simulink model "simulation_prev"  (R2021b)
settings: Solver=ode45  StartTime=0.0  StopTime=20.0  RelTol=1e-3
model workspace (MAT data in the model file):
  instants = 1
values from neighbouring files (symbols this model uses):
  c = modNE(x2,x2,e0,m,I,A,pc)    [ct_dynamics.m]    (also in dynamic_model_3R_spatial.m = [c1;c2;c3]; dynamic_model_simulation.m = [0.4; 0.2; 0.7]; run_experiment.m = [0.4; 0.2; 0.7])
  c0bar = norm(get_c_factorization_matrix(sol(1),sol(2),sol(3),sol(4),sol(5)))/norm(sol(3:5))    [compute_vel_obs_gain.m]    (also in dynamic_model_simulation.m = 1.96239028072; red_obs_gain_computation.m = c0; run_experiment.m = 1.96239028072)
  DHTABLE = [ pi/2      0         l(1)     q1 ... (first row only)    [compute_vel_obs_gain.m]    (also in dynamic_model_3R_spatial.m = [ pi/2      0      sym('L1') sym('q1'); dynamic_model_simulation.m = [ pi/2      0         l(1)     0; red_obs_gain_computation.m = [ pi/2      0         l(1)     0; run_experiment.m = [ pi/2      0         l(1)     0)
  eta = 1    [compute_vel_obs_gain.m]    (also in dynamic_model_simulation.m; red_obs_gain_computation.m; run_experiment.m)
  g0 = 9.81    [compute_vel_obs_gain.m]    (also in dynamic_model_3R_spatial.m; dynamic_model_simulation.m; modNE.m = 0; red_obs_gain_computation.m)
  I = zeros(3,3,N)    [compute_vel_obs_gain.m]    (also in dynamic_model_simulation.m; red_obs_gain_computation.m; run_experiment.m; run_simulation.m = zeros(3,3,3))
  K0 = c0bar*(v_max+eta)/(2*lambda_1)    [compute_vel_obs_gain.m]    (also in dynamic_model_simulation.m = 31.0539244645; red_obs_gain_computation.m = 0; run_experiment.m = 103.513081548)
  Kd = 3e1    (= 30)    [dynamic_model_simulation.m]    (also in run_experiment.m = 70; run_simulation.m = 10)
  Ko = 5e1    (= 50)    [dynamic_model_simulation.m]    (also in run_experiment.m; run_simulation.m = 0.1)
  Kp = 3e2    (= 300)    [dynamic_model_simulation.m]    (also in run_experiment.m = 70; run_simulation.m = 50)
  l = [0.5 0.5 0.4]'    [compute_eeJacobian.m]    (also in compute_vel_obs_gain.m; dynamic_model_simulation.m; eeJacobian_3R_spatial.m; red_obs_gain_computation.m)
  lambda_1 = min(min_first,min_third)/2    [compute_vel_obs_gain.m]    (also in dynamic_model_simulation.m = 0.0947894822263; red_obs_gain_computation.m = min_eig/2; run_experiment.m = 0.0473947411131)
  m = [15 10 5]'    [compute_vel_obs_gain.m]    (also in dynamic_model_simulation.m; red_obs_gain_computation.m; run_experiment.m; run_simulation.m = [m1 m2 m3]')
  pc = [0             -l(2)+dc(2) -l(3)+dc(3) ... (first row only)    [compute_vel_obs_gain.m]    (also in dynamic_model_simulation.m; red_obs_gain_computation.m; run_experiment.m)
  q0 = inverse_kinematics(p_init,l,soln_type)    [dynamic_model_simulation.m]    (also in run_experiment.m; run_simulation.m = [0,0,0]')
  r_c = 0.3    [dynamic_model_simulation.m]    (also in run_experiment.m)
  s0 = ceil(norm(dq0)/vbar)    [dynamic_model_simulation.m]
  T = simplify(T)    [DHMatrix.m]    (also in DHMatrix_sym.m; dynamic_model_3R_spatial.m = simplify(T1+T2+T3); dynamic_model_simulation.m = 2; run_experiment.m = 2)
  t0 = 2    [dynamic_model_simulation.m]    (also in run_experiment.m)
  T0 = 0.5*x2hat0'*M0*x2hat0    [dynamic_model_simulation.m]    (also in run_experiment.m)
  vbar = 2*eta+1    (= 3)    [dynamic_model_simulation.m]
  x0 = [pi/4,pi/4,1,1,1]'    [compute_vel_obs_gain.m]    (also in dynamic_model_simulation.m = [q0; dq0]; find_c0.m; run_experiment.m = [q0; dq0])
  z0 = [0 0 1]'    [dynamic_model_3R_spatial.m]    (also in dynamic_model_simulation.m = x2hat0 - K0*q0; run_experiment.m = x2hat0 - K0*q0)
undefined symbols (not defined in the file or in its folder): Levenberg, Marquardt, p_f, p_i, t_fin, t_init, time_int, trvec2tform
libraries: robotcorelib x3, SignalEditorBlockLib x1, robotmaniplib x1, matrix_library x1
(part 2 of 2)

== matlab function simulation_prev/reduced observer implementation/energy residual/MATLAB Function5 ==
  data: arrays input; T output; A output
function [T, A] = DHMatrix(arrays)
% T = DHMatrix(arrays) takes as inputs:
%   -arrays: a n-vector of vectors composed like this: [alpha a d theta]
% and outputs:
%   -T: the product of all the matrices corresponding to each vector of arrays
% Remember that:
% cos(q1 + q2) = cos(q1)*cos(q2) - sin(q1)*sin(q2)
% sin(q1 + q2) = cos(q1)*sin(q2) + cos(q2)*sin(q1)
% making use of the simplify function these are converted automatically

    T = eye(4);
    nums = size(arrays);
    
    A = zeros(4,4,nums(1));
    
    for i = 1:nums(1)
        line = arrays(i, :);
        R = [cos(line(4)) -cos(line(1))*sin(line(4)) sin(line(1))*sin(line(4)) line(2)*cos(line(4));
             sin(line(4)) cos(line(1))*cos(line(4)) -sin(line(1))*cos(line(4)) line(2)*sin(line(4));
             0 sin(line(1)) cos(line(1)) line(3);
             0 0 0 1];
        A(:,:,i) = R;
        T = T * R;   
    end
end

== matlab function simulation_prev/reduced observer implementation/energy residual/MATLAB Function6 ==
  data: dq input; u output; v input; ddq input; m input; I input; A input; pc input; g0 input
function u = modNE(dq,v,ddq,m,I,A,pc,g0)
% Implementation of Modified Newton-Euler algorithm

n = size(dq,1);
% check dimension consistency
if ~(size(v,1)==n && size(ddq,1)==n && size(dq,2)==1 && ...
     size(v,2)==1 && size(ddq,2)==1 && size(m,1)==n && ...
     size(I,3)==n && size(A,3)==n && size(pc,2)==n) 
    disp("Inconsistent input arguments dimension")
    u = zeros(n,1);
    return
end

% initialization
R = A(1:3,1:3,:);
p = [R(:,:,1)'*A(1:3,4,1) R(:,:,2)'*A(1:3,4,2) R(:,:,3)'*A(1:3,4,3)];
w = zeros(3,n+1);
wa = zeros(3,n+1);
dw = zeros(3,n+1);
a = zeros(3,n+1)-[[0 0 -g0]' zeros(3,n)];
ac = zeros(3,n+1);
f = zeros(3,n+1);
t = zeros(3,n+1);
u = zeros(n,1);

% forward recursion
for i = 2:n+1
   w(:,i) = R(:,:,i-1)'*(w(:,i-1)+dq(i-1)*[0 0 1]');
   wa(:,i) = R(:,:,i-1)'*(wa(:,i-1)+v(i-1)*[0 0 1]');
   dw(:,i) = R(:,:,i-1)'*(dw(:,i-1)+ddq(i-1)*[0 0 1]'+cross(dq(i-1)*wa(:,i-1),[0 0 1]'));
   a(:,i) = R(:,:,i-1)'*a(:,i-1)+cross(dw(:,i),p(:,i-1))+cross(w(:,i),cross(wa(:,i),p(:,i-1)));
   ac(:,i) = a(:,i)+cross(dw(:,i),pc(:,i-1))+cross(w(:,i),cross(wa(:,i),pc(:,i-1)));
end

w = w(:,2:n+1);
wa = wa(:,2:n+1);
dw = dw(:,2:n+1);
ac = ac(:,2:n+1);
R = cat(3,R,eye(3));

% backward recursion
for i = n:-1:1
    f(:,i) = R(:,:,i+1)*f(:,i+1)+m(i)*ac(:,i);
    t(:,i) = R(:,:,i+1)*t(:,i+1)+cross(R(:,:,i+1)*f(:,i+1),pc(:,i))-cross(f(:,i),p(:,i)+pc(:,i))+I(:,:,i)*dw(:,i)+cross(w(:,i),I(:,:,i)*wa(:,i));
    % assuming all revolute joints
    u(i) = t(:,i)'*(R(:,:,i)'*[0 0 1]');
end
end

== matlab function simulation_prev/reduced observer implementation/observer dynamics/MATLAB Function1 ==
  data: x2hat input; s input; vbar input; eta input; next_s output
function next_s = s_dynamics(x2hat,s,vbar,eta)
norm_x2hat = norm(x2hat);
if ((norm_x2hat >= s*vbar-eta) && ~(norm_x2hat <= s*vbar+eta))
    next_s = s+1;
elseif ((norm_x2hat <= (s-1)*vbar+eta) && ~(norm_x2hat >= (s-1)*vbar-eta) && s~=1)
    next_s = s-1;
else
    next_s = s;
end
end

== matlab function simulation_prev/finite differentiation/Controller/MATLAB Function1 ==
  data: dq input; u output; v input; ddq input; m input; I input; A input; pc input; g0 input
function u = modNE(dq,v,ddq,m,I,A,pc,g0)
% Implementation of Modified Newton-Euler algorithm

n = size(dq,1);
% check dimension consistency
if ~(size(v,1)==n && size(ddq,1)==n && size(dq,2)==1 && ...
     size(v,2)==1 && size(ddq,2)==1 && size(m,1)==n && ...
     size(I,3)==n && size(A,3)==n && size(pc,2)==n) 
    disp("Inconsistent input arguments dimension")
    u = zeros(n,1);
    return
end

% initialization
R = A(1:3,1:3,:);
p = [R(:,:,1)'*A(1:3,4,1) R(:,:,2)'*A(1:3,4,2) R(:,:,3)'*A(1:3,4,3)];
w = zeros(3,n+1);
wa = zeros(3,n+1);
dw = zeros(3,n+1);
a = zeros(3,n+1)-[[0 0 -g0]' zeros(3,n)];
ac = zeros(3,n+1);
f = zeros(3,n+1);
t = zeros(3,n+1);
u = zeros(n,1);

% forward recursion
for i = 2:n+1
   w(:,i) = R(:,:,i-1)'*(w(:,i-1)+dq(i-1)*[0 0 1]');
   wa(:,i) = R(:,:,i-1)'*(wa(:,i-1)+v(i-1)*[0 0 1]');
   dw(:,i) = R(:,:,i-1)'*(dw(:,i-1)+ddq(i-1)*[0 0 1]'+cross(dq(i-1)*wa(:,i-1),[0 0 1]'));
   a(:,i) = R(:,:,i-1)'*a(:,i-1)+cross(dw(:,i),p(:,i-1))+cross(w(:,i),cross(wa(:,i),p(:,i-1)));
   ac(:,i) = a(:,i)+cross(dw(:,i),pc(:,i-1))+cross(w(:,i),cross(wa(:,i),pc(:,i-1)));
end

w = w(:,2:n+1);
wa = wa(:,2:n+1);
dw = dw(:,2:n+1);
ac = ac(:,2:n+1);
R = cat(3,R,eye(3));

% backward recursion
for i = n:-1:1
    f(:,i) = R(:,:,i+1)*f(:,i+1)+m(i)*ac(:,i);
    t(:,i) = R(:,:,i+1)*t(:,i+1)+cross(R(:,:,i+1)*f(:,i+1),pc(:,i))-cross(f(:,i),p(:,i)+pc(:,i))+I(:,:,i)*dw(:,i)+cross(w(:,i),I(:,:,i)*wa(:,i));
    % assuming all revolute joints
    u(i) = t(:,i)'*(R(:,:,i)'*[0 0 1]');
end
end

== matlab function simulation_prev/finite differentiation/Controller/MATLAB Function3 ==
  data: arrays input; T output; A output
function [T, A] = DHMatrix(arrays)
% T = DHMatrix(arrays) takes as inputs:
%   -arrays: a n-vector of vectors composed like this: [alpha a d theta]
% and outputs:
%   -T: the product of all the matrices corresponding to each vector of arrays
% Remember that:
% cos(q1 + q2) = cos(q1)*cos(q2) - sin(q1)*sin(q2)
% sin(q1 + q2) = cos(q1)*sin(q2) + cos(q2)*sin(q1)
% making use of the simplify function these are converted automatically

    T = eye(4);
    nums = size(arrays);
    
    A = zeros(4,4,nums(1));
    
    for i = 1:nums(1)
        line = arrays(i, :);
        R = [cos(line(4)) -cos(line(1))*sin(line(4)) sin(line(1))*sin(line(4)) line(2)*cos(line(4));
             sin(line(4)) cos(line(1))*cos(line(4)) -sin(line(1))*cos(line(4)) line(2)*sin(line(4));
             0 sin(line(1)) cos(line(1)) line(3);
             0 0 0 1];
        A(:,:,i) = R;
        T = T * R;   
    end
end

== matlab function simulation_prev/finite differentiation/Robot dynamics/MATLAB Function ==
  data: x input; u input; dx output; m input; I input; A input; pc input; g0 input
function dx = ct_dynamics(x,u,m,I,A,pc,g0)
% return the continuous time dynamics given state and input
e0 = zeros(3,1);
e1 = [1 0 0]';
e2 = [0 1 0]';
e3 = [0 0 1]';
x2 = x(4:6);
%get inertia matrix M from modNE algorithm
M = [modNE(e0,e0,e1,m,I,A,pc,0) modNE(e0,e0,e2,m,I,A,pc,0) modNE(e0,e0,e3,m,I,A,pc,0)];
iM = inv(M);
cg =  modNE(x2,x2,e0,m,I,A,pc,g0);
dx=[x2;
    iM*(-cg+u)];
end

== matlab function simulation_prev/finite differentiation/Robot dynamics/MATLAB Function2 ==
  data: arrays input; T output; A output
function [T, A] = DHMatrix(arrays)
% T = DHMatrix(arrays) takes as inputs:
%   -arrays: a n-vector of vectors composed like this: [alpha a d theta]
% and outputs:
%   -T: the product of all the matrices corresponding to each vector of arrays
% Remember that:
% cos(q1 + q2) = cos(q1)*cos(q2) - sin(q1)*sin(q2)
% sin(q1 + q2) = cos(q1)*sin(q2) + cos(q2)*sin(q1)
% making use of the simplify function these are converted automatically

    T = eye(4);
    nums = size(arrays);
    
    A = zeros(4,4,nums(1));
    
    for i = 1:nums(1)
        line = arrays(i, :);
        R = [cos(line(4)) -cos(line(1))*sin(line(4)) sin(line(1))*sin(line(4)) line(2)*cos(line(4));
             sin(line(4)) cos(line(1))*cos(line(4)) -sin(line(1))*cos(line(4)) line(2)*sin(line(4));
             0 sin(line(1)) cos(line(1)) line(3);
             0 0 0 1];
        A(:,:,i) = R;
        T = T * R;   
    end
end

== matlab function simulation_prev/full state implementation/Robot dynamics/MATLAB Function ==
  data: x input; u input; dx output; m input; I input; A input; pc input; g0 input
function dx = ct_dynamics(x,u,m,I,A,pc,g0)
% return the continuous time dynamics given state and input
e0 = zeros(3,1);
e1 = [1 0 0]';
e2 = [0 1 0]';
e3 = [0 0 1]';
x2 = x(4:6);
%get inertia matrix M from modNE algorithm
M = [modNE(e0,e0,e1,m,I,A,pc,0) modNE(e0,e0,e2,m,I,A,pc,0) modNE(e0,e0,e3,m,I,A,pc,0)];
cg =  modNE(x2,x2,e0,m,I,A,pc,g0);
dx=[x2;
    inv(M)*(-cg+u)];
end

== matlab function simulation_prev/finite differentiation/energy residual/MATLAB Function2 ==
  data: dq input; u output; v input; ddq input; m input; I input; A input; pc input; g0 input
function u = modNE(dq,v,ddq,m,I,A,pc,g0)
% Implementation of Modified Newton-Euler algorithm

n = size(dq,1);
% check dimension consistency
if ~(size(v,1)==n && size(ddq,1)==n && size(dq,2)==1 && ...
     size(v,2)==1 && size(ddq,2)==1 && size(m,1)==n && ...
     size(I,3)==n && size(A,3)==n && size(pc,2)==n) 
    disp("Inconsistent input arguments dimension")
    u = zeros(n,1);
    return
end

% initialization
R = A(1:3,1:3,:);
p = [R(:,:,1)'*A(1:3,4,1) R(:,:,2)'*A(1:3,4,2) R(:,:,3)'*A(1:3,4,3)];
w = zeros(3,n+1);
wa = zeros(3,n+1);
dw = zeros(3,n+1);
a = zeros(3,n+1)-[[0 0 -g0]' zeros(3,n)];
ac = zeros(3,n+1);
f = zeros(3,n+1);
t = zeros(3,n+1);
u = zeros(n,1);

% forward recursion
for i = 2:n+1
   w(:,i) = R(:,:,i-1)'*(w(:,i-1)+dq(i-1)*[0 0 1]');
   wa(:,i) = R(:,:,i-1)'*(wa(:,i-1)+v(i-1)*[0 0 1]');
   dw(:,i) = R(:,:,i-1)'*(dw(:,i-1)+ddq(i-1)*[0 0 1]'+cross(dq(i-1)*wa(:,i-1),[0 0 1]'));
   a(:,i) = R(:,:,i-1)'*a(:,i-1)+cross(dw(:,i),p(:,i-1))+cross(w(:,i),cross(wa(:,i),p(:,i-1)));
   ac(:,i) = a(:,i)+cross(dw(:,i),pc(:,i-1))+cross(w(:,i),cross(wa(:,i),pc(:,i-1)));
end

w = w(:,2:n+1);
wa = wa(:,2:n+1);
dw = dw(:,2:n+1);
ac = ac(:,2:n+1);
R = cat(3,R,eye(3));

% backward recursion
for i = n:-1:1
    f(:,i) = R(:,:,i+1)*f(:,i+1)+m(i)*ac(:,i);
    t(:,i) = R(:,:,i+1)*t(:,i+1)+cross(R(:,:,i+1)*f(:,i+1),pc(:,i))-cross(f(:,i),p(:,i)+pc(:,i))+I(:,:,i)*dw(:,i)+cross(w(:,i),I(:,:,i)*wa(:,i));
    % assuming all revolute joints
    u(i) = t(:,i)'*(R(:,:,i)'*[0 0 1]');
end
end

== matlab function simulation_prev/finite differentiation/energy residual/MATLAB Function3 ==
  data: dq input; u output; v input; ddq input; m input; I input; A input; pc input; g0 input
function u = modNE(dq,v,ddq,m,I,A,pc,g0)
% Implementation of Modified Newton-Euler algorithm

n = size(dq,1);
% check dimension consistency
if ~(size(v,1)==n && size(ddq,1)==n && size(dq,2)==1 && ...
     size(v,2)==1 && size(ddq,2)==1 && size(m,1)==n && ...
     size(I,3)==n && size(A,3)==n && size(pc,2)==n) 
    disp("Inconsistent input arguments dimension")
    u = zeros(n,1);
    return
end

% initialization
R = A(1:3,1:3,:);
p = [R(:,:,1)'*A(1:3,4,1) R(:,:,2)'*A(1:3,4,2) R(:,:,3)'*A(1:3,4,3)];
w = zeros(3,n+1);
wa = zeros(3,n+1);
dw = zeros(3,n+1);
a = zeros(3,n+1)-[[0 0 -g0]' zeros(3,n)];
ac = zeros(3,n+1);
f = zeros(3,n+1);
t = zeros(3,n+1);
u = zeros(n,1);

% forward recursion
for i = 2:n+1
   w(:,i) = R(:,:,i-1)'*(w(:,i-1)+dq(i-1)*[0 0 1]');
   wa(:,i) = R(:,:,i-1)'*(wa(:,i-1)+v(i-1)*[0 0 1]');
   dw(:,i) = R(:,:,i-1)'*(dw(:,i-1)+ddq(i-1)*[0 0 1]'+cross(dq(i-1)*wa(:,i-1),[0 0 1]'));
   a(:,i) = R(:,:,i-1)'*a(:,i-1)+cross(dw(:,i),p(:,i-1))+cross(w(:,i),cross(wa(:,i),p(:,i-1)));
   ac(:,i) = a(:,i)+cross(dw(:,i),pc(:,i-1))+cross(w(:,i),cross(wa(:,i),pc(:,i-1)));
end

w = w(:,2:n+1);
wa = wa(:,2:n+1);
dw = dw(:,2:n+1);
ac = ac(:,2:n+1);
R = cat(3,R,eye(3));

% backward recursion
for i = n:-1:1
    f(:,i) = R(:,:,i+1)*f(:,i+1)+m(i)*ac(:,i);
    t(:,i) = R(:,:,i+1)*t(:,i+1)+cross(R(:,:,i+1)*f(:,i+1),pc(:,i))-cross(f(:,i),p(:,i)+pc(:,i))+I(:,:,i)*dw(:,i)+cross(w(:,i),I(:,:,i)*wa(:,i));
    % assuming all revolute joints
    u(i) = t(:,i)'*(R(:,:,i)'*[0 0 1]');
end
end

== matlab function simulation_prev/finite differentiation/energy residual/MATLAB Function4 ==
  data: dq input; u output; v input; ddq input; m input; I input; A input; pc input; g0 input
function u = modNE(dq,v,ddq,m,I,A,pc,g0)
% Implementation of Modified Newton-Euler algorithm

n = size(dq,1);
% check dimension consistency
if ~(size(v,1)==n && size(ddq,1)==n && size(dq,2)==1 && ...
     size(v,2)==1 && size(ddq,2)==1 && size(m,1)==n && ...
     size(I,3)==n && size(A,3)==n && size(pc,2)==n) 
    disp("Inconsistent input arguments dimension")
    u = zeros(n,1);
    return
end

% initialization
R = A(1:3,1:3,:);
p = [R(:,:,1)'*A(1:3,4,1) R(:,:,2)'*A(1:3,4,2) R(:,:,3)'*A(1:3,4,3)];
w = zeros(3,n+1);
wa = zeros(3,n+1);
dw = zeros(3,n+1);
a = zeros(3,n+1)-[[0 0 -g0]' zeros(3,n)];
ac = zeros(3,n+1);
f = zeros(3,n+1);
t = zeros(3,n+1);
u = zeros(n,1);

% forward recursion
for i = 2:n+1
   w(:,i) = R(:,:,i-1)'*(w(:,i-1)+dq(i-1)*[0 0 1]');
   wa(:,i) = R(:,:,i-1)'*(wa(:,i-1)+v(i-1)*[0 0 1]');
   dw(:,i) = R(:,:,i-1)'*(dw(:,i-1)+ddq(i-1)*[0 0 1]'+cross(dq(i-1)*wa(:,i-1),[0 0 1]'));
   a(:,i) = R(:,:,i-1)'*a(:,i-1)+cross(dw(:,i),p(:,i-1))+cross(w(:,i),cross(wa(:,i),p(:,i-1)));
   ac(:,i) = a(:,i)+cross(dw(:,i),pc(:,i-1))+cross(w(:,i),cross(wa(:,i),pc(:,i-1)));
end

w = w(:,2:n+1);
wa = wa(:,2:n+1);
dw = dw(:,2:n+1);
ac = ac(:,2:n+1);
R = cat(3,R,eye(3));

% backward recursion
for i = n:-1:1
    f(:,i) = R(:,:,i+1)*f(:,i+1)+m(i)*ac(:,i);
    t(:,i) = R(:,:,i+1)*t(:,i+1)+cross(R(:,:,i+1)*f(:,i+1),pc(:,i))-cross(f(:,i),p(:,i)+pc(:,i))+I(:,:,i)*dw(:,i)+cross(w(:,i),I(:,:,i)*wa(:,i));
    % assuming all revolute joints
    u(i) = t(:,i)'*(R(:,:,i)'*[0 0 1]');
end
end

== matlab function simulation_prev/finite differentiation/energy residual/MATLAB Function5 ==
  data: arrays input; T output; A output
function [T, A] = DHMatrix(arrays)
% T = DHMatrix(arrays) takes as inputs:
%   -arrays: a n-vector of vectors composed like this: [alpha a d theta]
% and outputs:
%   -T: the product of all the matrices corresponding to each vector of arrays
% Remember that:
% cos(q1 + q2) = cos(q1)*cos(q2) - sin(q1)*sin(q2)
% sin(q1 + q2) = cos(q1)*sin(q2) + cos(q2)*sin(q1)
% making use of the simplify function these are converted automatically

    T = eye(4);
    nums = size(arrays);
    
    A = zeros(4,4,nums(1));
    
    for i = 1:nums(1)
        line = arrays(i, :);
        R = [cos(line(4)) -cos(line(1))*sin(line(4)) sin(line(1))*sin(line(4)) line(2)*cos(line(4));
             sin(line(4)) cos(line(1))*cos(line(4)) -sin(line(1))*cos(line(4)) line(2)*sin(line(4));
             0 sin(line(1)) cos(line(1)) line(3);
             0 0 0 1];
        A(:,:,i) = R;
        T = T * R;   
    end
end

== matlab function simulation_prev/finite differentiation/energy residual/MATLAB Function6 ==
  data: dq input; u output; v input; ddq input; m input; I input; A input; pc input; g0 input
function u = modNE(dq,v,ddq,m,I,A,pc,g0)
% Implementation of Modified Newton-Euler algorithm

n = size(dq,1);
% check dimension consistency
if ~(size(v,1)==n && size(ddq,1)==n && size(dq,2)==1 && ...
     size(v,2)==1 && size(ddq,2)==1 && size(m,1)==n && ...
     size(I,3)==n && size(A,3)==n && size(pc,2)==n) 
    disp("Inconsistent input arguments dimension")
    u = zeros(n,1);
    return
end

% initialization
R = A(1:3,1:3,:);
p = [R(:,:,1)'*A(1:3,4,1) R(:,:,2)'*A(1:3,4,2) R(:,:,3)'*A(1:3,4,3)];
w = zeros(3,n+1);
wa = zeros(3,n+1);
dw = zeros(3,n+1);
a = zeros(3,n+1)-[[0 0 -g0]' zeros(3,n)];
ac = zeros(3,n+1);
f = zeros(3,n+1);
t = zeros(3,n+1);
u = zeros(n,1);

% forward recursion
for i = 2:n+1
   w(:,i) = R(:,:,i-1)'*(w(:,i-1)+dq(i-1)*[0 0 1]');
   wa(:,i) = R(:,:,i-1)'*(wa(:,i-1)+v(i-1)*[0 0 1]');
   dw(:,i) = R(:,:,i-1)'*(dw(:,i-1)+ddq(i-1)*[0 0 1]'+cross(dq(i-1)*wa(:,i-1),[0 0 1]'));
   a(:,i) = R(:,:,i-1)'*a(:,i-1)+cross(dw(:,i),p(:,i-1))+cross(w(:,i),cross(wa(:,i),p(:,i-1)));
   ac(:,i) = a(:,i)+cross(dw(:,i),pc(:,i-1))+cross(w(:,i),cross(wa(:,i),pc(:,i-1)));
end

w = w(:,2:n+1);
wa = wa(:,2:n+1);
dw = dw(:,2:n+1);
ac = ac(:,2:n+1);
R = cat(3,R,eye(3));

% backward recursion
for i = n:-1:1
    f(:,i) = R(:,:,i+1)*f(:,i+1)+m(i)*ac(:,i);
    t(:,i) = R(:,:,i+1)*t(:,i+1)+cross(R(:,:,i+1)*f(:,i+1),pc(:,i))-cross(f(:,i),p(:,i)+pc(:,i))+I(:,:,i)*dw(:,i)+cross(w(:,i),I(:,:,i)*wa(:,i));
    % assuming all revolute joints
    u(i) = t(:,i)'*(R(:,:,i)'*[0 0 1]');
end
end

== matlab function simulation_prev/Trajectory generator/MATLAB Function ==
  data: q input; dq output; dx input; ddx input; ddq output
function [dq,ddq] = inv_diff_kin(q,dx,ddx)
Jee = get_Jee(q(1),q(2),q(3));
dq = pinv(Jee)*dx;
dJee = get_dJee(q(1),q(2),q(3),dq(1),dq(2),dq(3));
ddq = pinv(Jee)*(ddx-dJee*dq);
end

== matlab function simulation_prev/full state implementation/Robot dynamics/MATLAB Function2 ==
  data: arrays input; T output; A output
function [T, A] = DHMatrix(arrays)
% T = DHMatrix(arrays) takes as inputs:
%   -arrays: a n-vector of vectors composed like this: [alpha a d theta]
% and outputs:
%   -T: the product of all the matrices corresponding to each vector of arrays
% Remember that:
% cos(q1 + q2) = cos(q1)*cos(q2) - sin(q1)*sin(q2)
% sin(q1 + q2) = cos(q1)*sin(q2) + cos(q2)*sin(q1)
% making use of the simplify function these are converted automatically

    T = eye(4);
    nums = size(arrays);
    
    A = zeros(4,4,nums(1));
    
    for i = 1:nums(1)
        line = arrays(i, :);
        R = [cos(line(4)) -cos(line(1))*sin(line(4)) sin(line(1))*sin(line(4)) line(2)*cos(line(4));
             sin(line(4)) cos(line(1))*cos(line(4)) -sin(line(1))*cos(line(4)) line(2)*sin(line(4));
             0 sin(line(1)) cos(line(1)) line(3);
             0 0 0 1];
        A(:,:,i) = R;
        T = T * R;   
    end
end

== matlab function simulation_prev/full state implementation/Controller/MATLAB Function3 ==
  data: arrays input; T output; A output
function [T, A] = DHMatrix(arrays)
% T = DHMatrix(arrays) takes as inputs:
%   -arrays: a n-vector of vectors composed like this: [alpha a d theta]
% and outputs:
%   -T: the product of all the matrices corresponding to each vector of arrays
% Remember that:
% cos(q1 + q2) = cos(q1)*cos(q2) - sin(q1)*sin(q2)
% sin(q1 + q2) = cos(q1)*sin(q2) + cos(q2)*sin(q1)
% making use of the simplify function these are converted automatically

    T = eye(4);
    nums = size(arrays);
    
    A = zeros(4,4,nums(1));
    
    for i = 1:nums(1)
        line = arrays(i, :);
        R = [cos(line(4)) -cos(line(1))*sin(line(4)) sin(line(1))*sin(line(4)) line(2)*cos(line(4));
             sin(line(4)) cos(line(1))*cos(line(4)) -sin(line(1))*cos(line(4)) line(2)*sin(line(4));
             0 sin(line(1)) cos(line(1)) line(3);
             0 0 0 1];
        A(:,:,i) = R;
        T = T * R;   
    end
end

== matlab function simulation_prev/external torque generator/MATLAB Function ==
  data: q input; J output; l input
function J = eeJacobian(q,l)
J = [-sin(q(1))*(l(3)*cos(q(2)+q(3))+l(2)*cos(q(2)))    -cos(q(1))*(l(3)*sin(q(2)+q(3))+l(2)*sin(q(2))) -l(3)*sin(q(2)+q(3))*cos(q(1));
     cos(q(1))*(l(3)*cos(q(2)+q(3))+l(2)*cos(q(2)))     -sin(q(1))*(l(3)*sin(q(2)+q(3))+l(2)*sin(q(2))) -l(3)*sin(q(2)+q(3))*sin(q(1));
     0                                                  l(3)*cos(q(2)+q(3))+l(2)*cos(q(2))              l(3)*cos(q(2)+q(3))];

== matlab function simulation_prev/full state implementation/energy residual/MATLAB Function2 ==
  data: dq input; u output; v input; ddq input; m input; I input; A input; pc input; g0 input
function u = modNE(dq,v,ddq,m,I,A,pc,g0)
% Implementation of Modified Newton-Euler algorithm

n = size(dq,1);
% check dimension consistency
if ~(size(v,1)==n && size(ddq,1)==n && size(dq,2)==1 && ...
     size(v,2)==1 && size(ddq,2)==1 && size(m,1)==n && ...
     size(I,3)==n && size(A,3)==n && size(pc,2)==n) 
    disp("Inconsistent input arguments dimension")
    u = zeros(n,1);
    return
end

% initialization
R = A(1:3,1:3,:);
p = [R(:,:,1)'*A(1:3,4,1) R(:,:,2)'*A(1:3,4,2) R(:,:,3)'*A(1:3,4,3)];
w = zeros(3,n+1);
wa = zeros(3,n+1);
dw = zeros(3,n+1);
a = zeros(3,n+1)-[[0 0 -g0]' zeros(3,n)];
ac = zeros(3,n+1);
f = zeros(3,n+1);
t = zeros(3,n+1);
u = zeros(n,1);

% forward recursion
for i = 2:n+1
   w(:,i) = R(:,:,i-1)'*(w(:,i-1)+dq(i-1)*[0 0 1]');
   wa(:,i) = R(:,:,i-1)'*(wa(:,i-1)+v(i-1)*[0 0 1]');
   dw(:,i) = R(:,:,i-1)'*(dw(:,i-1)+ddq(i-1)*[0 0 1]'+cross(dq(i-1)*wa(:,i-1),[0 0 1]'));
   a(:,i) = R(:,:,i-1)'*a(:,i-1)+cross(dw(:,i),p(:,i-1))+cross(w(:,i),cross(wa(:,i),p(:,i-1)));
   ac(:,i) = a(:,i)+cross(dw(:,i),pc(:,i-1))+cross(w(:,i),cross(wa(:,i),pc(:,i-1)));
end

w = w(:,2:n+1);
wa = wa(:,2:n+1);
dw = dw(:,2:n+1);
ac = ac(:,2:n+1);
R = cat(3,R,eye(3));

% backward recursion
for i = n:-1:1
    f(:,i) = R(:,:,i+1)*f(:,i+1)+m(i)*ac(:,i);
    t(:,i) = R(:,:,i+1)*t(:,i+1)+cross(R(:,:,i+1)*f(:,i+1),pc(:,i))-cross(f(:,i),p(:,i)+pc(:,i))+I(:,:,i)*dw(:,i)+cross(w(:,i),I(:,:,i)*wa(:,i));
    % assuming all revolute joints
    u(i) = t(:,i)'*(R(:,:,i)'*[0 0 1]');
end
end

== matlab function simulation_prev/full state implementation/energy residual/MATLAB Function3 ==
  data: dq input; u output; v input; ddq input; m input; I input; A input; pc input; g0 input
function u = modNE(dq,v,ddq,m,I,A,pc,g0)
% Implementation of Modified Newton-Euler algorithm

n = size(dq,1);
% check dimension consistency
if ~(size(v,1)==n && size(ddq,1)==n && size(dq,2)==1 && ...
     size(v,2)==1 && size(ddq,2)==1 && size(m,1)==n && ...
     size(I,3)==n && size(A,3)==n && size(pc,2)==n) 
    disp("Inconsistent input arguments dimension")
    u = zeros(n,1);
    return
end

% initialization
R = A(1:3,1:3,:);
p = [R(:,:,1)'*A(1:3,4,1) R(:,:,2)'*A(1:3,4,2) R(:,:,3)'*A(1:3,4,3)];
w = zeros(3,n+1);
wa = zeros(3,n+1);
dw = zeros(3,n+1);
a = zeros(3,n+1)-[[0 0 -g0]' zeros(3,n)];
ac = zeros(3,n+1);
f = zeros(3,n+1);
t = zeros(3,n+1);
u = zeros(n,1);

% forward recursion
for i = 2:n+1
   w(:,i) = R(:,:,i-1)'*(w(:,i-1)+dq(i-1)*[0 0 1]');
   wa(:,i) = R(:,:,i-1)'*(wa(:,i-1)+v(i-1)*[0 0 1]');
   dw(:,i) = R(:,:,i-1)'*(dw(:,i-1)+ddq(i-1)*[0 0 1]'+cross(dq(i-1)*wa(:,i-1),[0 0 1]'));
   a(:,i) = R(:,:,i-1)'*a(:,i-1)+cross(dw(:,i),p(:,i-1))+cross(w(:,i),cross(wa(:,i),p(:,i-1)));
   ac(:,i) = a(:,i)+cross(dw(:,i),pc(:,i-1))+cross(w(:,i),cross(wa(:,i),pc(:,i-1)));
end

w = w(:,2:n+1);
wa = wa(:,2:n+1);
dw = dw(:,2:n+1);
ac = ac(:,2:n+1);
R = cat(3,R,eye(3));

% backward recursion
for i = n:-1:1
    f(:,i) = R(:,:,i+1)*f(:,i+1)+m(i)*ac(:,i);
    t(:,i) = R(:,:,i+1)*t(:,i+1)+cross(R(:,:,i+1)*f(:,i+1),pc(:,i))-cross(f(:,i),p(:,i)+pc(:,i))+I(:,:,i)*dw(:,i)+cross(w(:,i),I(:,:,i)*wa(:,i));
    % assuming all revolute joints
    u(i) = t(:,i)'*(R(:,:,i)'*[0 0 1]');
end
end

== matlab function simulation_prev/full state implementation/energy residual/MATLAB Function4 ==
  data: dq input; u output; v input; ddq input; m input; I input; A input; pc input; g0 input
function u = modNE(dq,v,ddq,m,I,A,pc,g0)
% Implementation of Modified Newton-Euler algorithm

n = size(dq,1);
% check dimension consistency
if ~(size(v,1)==n && size(ddq,1)==n && size(dq,2)==1 && ...
     size(v,2)==1 && size(ddq,2)==1 && size(m,1)==n && ...
     size(I,3)==n && size(A,3)==n && size(pc,2)==n) 
    disp("Inconsistent input arguments dimension")
    u = zeros(n,1);
    return
end

% initialization
R = A(1:3,1:3,:);
p = [R(:,:,1)'*A(1:3,4,1) R(:,:,2)'*A(1:3,4,2) R(:,:,3)'*A(1:3,4,3)];
w = zeros(3,n+1);
wa = zeros(3,n+1);
dw = zeros(3,n+1);
a = zeros(3,n+1)-[[0 0 -g0]' zeros(3,n)];
ac = zeros(3,n+1);
f = zeros(3,n+1);
t = zeros(3,n+1);
u = zeros(n,1);

% forward recursion
for i = 2:n+1
   w(:,i) = R(:,:,i-1)'*(w(:,i-1)+dq(i-1)*[0 0 1]');
   wa(:,i) = R(:,:,i-1)'*(wa(:,i-1)+v(i-1)*[0 0 1]');
   dw(:,i) = R(:,:,i-1)'*(dw(:,i-1)+ddq(i-1)*[0 0 1]'+cross(dq(i-1)*wa(:,i-1),[0 0 1]'));
   a(:,i) = R(:,:,i-1)'*a(:,i-1)+cross(dw(:,i),p(:,i-1))+cross(w(:,i),cross(wa(:,i),p(:,i-1)));
   ac(:,i) = a(:,i)+cross(dw(:,i),pc(:,i-1))+cross(w(:,i),cross(wa(:,i),pc(:,i-1)));
end

w = w(:,2:n+1);
wa = wa(:,2:n+1);
dw = dw(:,2:n+1);
ac = ac(:,2:n+1);
R = cat(3,R,eye(3));

% backward recursion
for i = n:-1:1
    f(:,i) = R(:,:,i+1)*f(:,i+1)+m(i)*ac(:,i);
    t(:,i) = R(:,:,i+1)*t(:,i+1)+cross(R(:,:,i+1)*f(:,i+1),pc(:,i))-cross(f(:,i),p(:,i)+pc(:,i))+I(:,:,i)*dw(:,i)+cross(w(:,i),I(:,:,i)*wa(:,i));
    % assuming all revolute joints
    u(i) = t(:,i)'*(R(:,:,i)'*[0 0 1]');
end
end
